simulink model "tempregler_modell"  (R2024a)
settings: Solver=VariableStepAuto  StartTime=0.0  StopTime=4200  RelTol=1e-3
values from neighbouring files (symbols this model uses):
  controller_off = -0.01    [tempregler.m]
  controlller_on = 0.01    [tempregler.m]
  k1 = 10/400    (= 0.025)    [tempregler.m]
  k2 = 400/230    (= 1.73913043478)    [tempregler.m]
  time_const = 15*60    (= 900)    [tempregler.m]
settings Model: Creator=janho  LastModifiedBy=janho

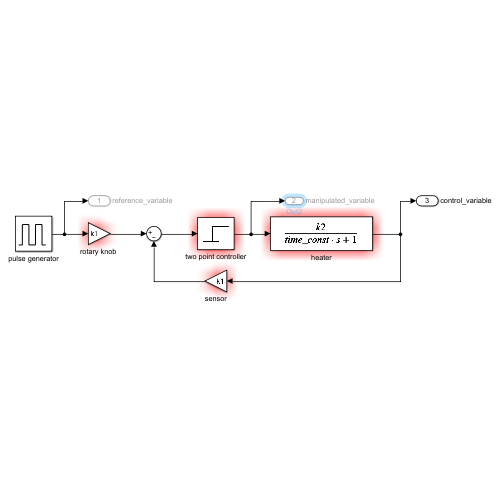
[thumbnail: Simulink's stored preview of the top-level diagram]
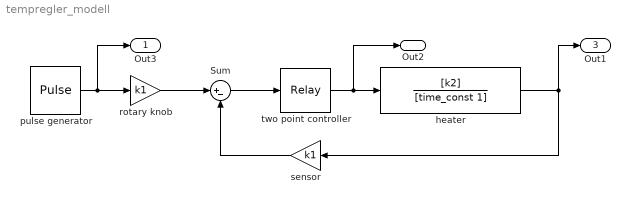
== system tempregler_modell ==
  Sum : Sum  Inputs=|+-
  heater : TransferFcn  Numerator=[k2]  Denominator=[time_const 1]
  pulse generator : DiscretePulseGenerator  PulseType=Time based  Amplitude=160  Period=70*60  PulseWidth=30 / 70 * 100
  "rotary knob " : Gain  Gain=k1
  sensor : Gain  Gain=k1
  two point controller : Relay  OnSwitchValue=controlller_on  OffSwitchValue=controller_off  OnOutputValue=230  ZeroCross=off
  Out3 : Outport  SignalName=reference_variable  SampleTime=0  LockScale=on
      settings: VarSizeSig=Yes  EnsureOutportIsVirtual=on
  Out2 : Outport  Port=2  SignalName=manipulated_variable  LockScale=on
      settings: VarSizeSig=Yes  EnsureOutportIsVirtual=on
  Out1 : Outport  Port=3  SignalName=control_variable
  wires:
  two point controller/1 -> heater/1, Out2/1
  sensor/1 -> Sum/2
  "rotary knob "/1 -> Sum/1
  pulse generator/1 -> Out3/1, "rotary knob "/1
  Sum/1 -> two point controller/1
  heater/1 -> sensor/1, Out1/1
